simulink model "ModelProcessPID"  (R2018b)
settings: Solver=FixedStepAuto  StartTime=0.0  StopTime=150  RelTol=1e-3
model workspace (MAT data in the model file):
  tmLag1 = 10
  tmLag2 = 10
  tmLag3 = 5
settings Model: Creator=Backbone  LastModifiedBy=Siemens
settings DataIOCC: LimitDataPoints=on  SaveFormat=Array  SaveOutput=off  SaveTime=off
settings OptimizationCC: LifeSpan=1
settings DebuggingCC: AllowSymbolicDim=off  SFUnexpectedBacktrackingDiag=warning  SFNoUnconditionalDefaultTransitionDiag=warning
settings HardwareCC: ProdBitPerPointer=32  ProdBitPerSizeT=32  ProdBitPerPtrDiffT=32  ProdWordSize=32  ProdHWDeviceType=Intel->x86-32 (Windows32)
settings ModelReferenceCC: PropagateSignalLabelsOutOfModel=off
settings SFSimCC: SimUseLocalCustomCode=off
settings RTWCC: SystemTargetFile=Target_1500S_V1_0_grt.tlc  GenCodeOnly=on  GenerateMakefile=off  TemplateMakefile=Target_1500S_V1_0_grt.tmf  Description=Target for ODK capable S7-1500 Controllers based on Simulink Coder  RTWVerbose=off  RTWUseLocalCustomCode=off  TargetLang=C++
settings CodeAppCC: StateflowObjectComments=on
settings STFCustomTargetCC: ModelReferenceCompliant=off  CombineOutputUpdateFcns=on  SystemTargetFile=Target_1500S_V1_0_grt.tlc
settings GRTTargetCC: TargetLangStandard=C89/C90 (ANSI)  ModelReferenceCompliant=off  ParMdlRefBuildCompliant=off  CompOptLevelCompliant=off  ConcurrentExecutionCompliant=off  MatFileLogging=off  CPPClassGenCompliant=off  UseToolchainInfoCompliant=off  ExtModeStaticAlloc=on  ExtModeTransport=1  ExtModeMexFile=ext_comm_target1500s  ExtModeMexArgs='192.168.0.1'
settings ConfigComp: CovMetricSettings=dw  CovHtmlReporting=on  CovSaveCumulativeToWorkspaceVar=on  CovSaveSingleToWorkspaceVar=on  CovExternalEMLEnable=off

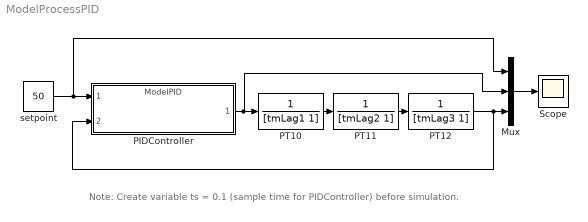
== system ModelProcessPID ==
  note: Note: Create variable ts = 0.1 (sample time for PIDController) before simulation.
  Mux : Mux  Inputs=3
  PIDController : ModelReference  ModelNameDialog=ModelPID.slx  SimulationMode=Normal  ModelReferenceVersion=1.115
  PT10 : TransferFcn  Denominator=[tmLag1 1]
  PT11 : TransferFcn  Denominator=[tmLag2 1]
  PT12 : TransferFcn  Denominator=[tmLag3 1]
  Scope : Scope
  setpoint : Constant  Value=50
  wires:
  PIDController/1 -> Mux/2, PT10/1
  setpoint/1 -> Mux/1, PIDController/1
  Mux/1 -> Scope/1
  PT12/1 -> PIDController/2, Mux/3
  PT10/1 -> PT11/1
  PT11/1 -> PT12/1
